simulink model "test3_4_model"  (R2018b)
settings: Solver=VariableStepAuto  StartTime=0.0  StopTime=Endtime  RelTol=1e-3
values from neighbouring files (symbols this model uses):
  C = M * c    (= 4187)    [test3_4.m]
  d0 = 20    [test3_4.m]
  q1 = 300    [test3_4.m]
  R = 0.1    [test3_4.m]
settings Model: Creator=nharada  LastModifiedBy=nharada

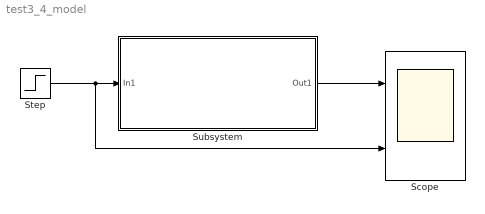
== system test3_4_model ==
  Scope : Scope  NumInputPorts=2
  Step : Step  Time=100  After=q1  SampleTime=0
  Subsystem : Subsystem
  wires:
  Subsystem/1(Out1) -> Scope/1
  Step/1 -> Scope/2, Subsystem/1(In1)

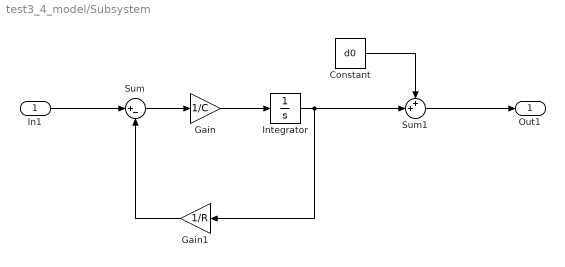
== system test3_4_model/Subsystem ==
  In1 : Inport
  Constant : Constant  Value=d0
  Gain : Gain  Gain=1/C
  Gain1 : Gain  Gain=1/R
  Integrator : Integrator
  Sum : Sum  Inputs=|+-
  Sum1 : Sum  Inputs=++|
  Out1 : Outport
  wires:
  Constant/1 -> Sum1/1
  Integrator/1 -> Sum1/2, Gain1/1
  Sum1/1 -> Out1/1
  Sum/1 -> Gain/1
  In1/1 -> Sum/1
  Gain1/1 -> Sum/2
  Gain/1 -> Integrator/1
